simulink model "ES205_lab_5_dual_model_orig"  (R2021a)
settings: Solver=VariableStepAuto  StartTime=0.0  StopTime=tf_double  MaxStep=maxstep  RelTol=tol  AbsTol=tol
values from neighbouring files (symbols this model uses):
  a1 = 3.49    [ES205_lab_5_script.m]
  a2 = 3.24    [ES205_lab_5_script.m]
  Aout1 = pi * (d1/2)^2    (= 0.0881413088873)    [ES205_lab_5_script.m]
  Aout2 = pi * (d2/2)^2    (= 0.0452389342117)    [ES205_lab_5_script.m]
  Atank1 = 22.94    [ES205_lab_5_script.m]
  Atank2 = 22.94    [ES205_lab_5_script.m]
  b2 = 0.5    [ES205_lab_5_script.m]
  Cd1_orig = 0.7    [ES205_lab_5_script.m]
  Cd2_orig = 0.7    [ES205_lab_5_script.m]
  g = 32.2 * 12    (= 386.4)    [ES205_lab_5_script.m]
  h1_0_double = h1data_double(1)    [ES205_lab_5_script.m]
  h2_0_double = h2data_double(2)    [ES205_lab_5_script.m]
settings Model: Creator=schimmer  LastModifiedBy=schimmer
settings DataIOCC: SaveOutput=off  SignalLogging=off  DSMLogging=off  SaveTime=off  ReturnWorkspaceOutputs=off  OutputOption=SpecifiedOutputTimes  OutputTimes=tdata_double

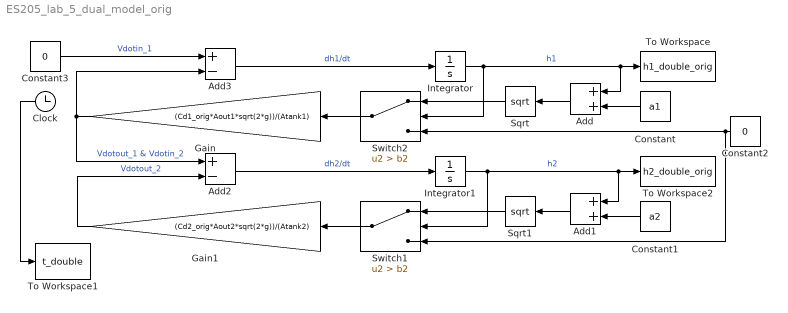
== system ES205_lab_5_dual_model_orig ==
  Add : Sum
  Add1 : Sum
  Add2 : Sum  Inputs=+-
  Add3 : Sum  Inputs=+-
  Clock : Clock
  Constant : Constant  Value=a1
  Constant1 : Constant  Value=a2
  Constant2 : Constant  Value=0
  Constant3 : Constant  Value=0
  Gain : Gain  Gain=(Cd1_orig*Aout1*sqrt(2*g))/(Atank1)
  Gain1 : Gain  Gain=(Cd2_orig*Aout2*sqrt(2*g))/(Atank2)
  Integrator : Integrator  InitialCondition=h1_0_double
  Integrator1 : Integrator  InitialCondition=h2_0_double
  Sqrt : Sqrt  SaturateOnIntegerOverflow=on
  Sqrt1 : Sqrt  SaturateOnIntegerOverflow=on
  Switch1 : Switch  Criteria=u2 > Threshold  Threshold=b2
  Switch2 : Switch  Criteria=u2 > Threshold  Threshold=b2
  To Workspace : ToWorkspace  VariableName=h1_double_orig  SampleTime=-1
  To Workspace1 : ToWorkspace  VariableName=t_double  SampleTime=-1
  To Workspace2 : ToWorkspace  VariableName=h2_double_orig  SampleTime=-1
  wires:
  Clock/1 -> To Workspace1/1
  Gain/1 -> Add2/1, Add3/2  "Vdotout_1 & Vdotin_2"
  Integrator/1 -> Add/1, To Workspace/1, Switch2/2  "h1"
  Sqrt/1 -> Switch2/1
  Add/1 -> Sqrt/1
  Constant/1 -> Add/2
  Constant1/1 -> Add1/2
  Integrator1/1 -> Switch1/2, Add1/1, To Workspace2/1  "h2"
  Add1/1 -> Sqrt1/1
  Switch2/1 -> Gain/1
  Add2/1 -> Integrator1/1  "dh2/dt"
  Sqrt1/1 -> Switch1/1
  Constant2/1 -> Switch1/3, Switch2/3
  Switch1/1 -> Gain1/1
  Constant3/1 -> Add3/1  "Vdotin_1"
  Add3/1 -> Integrator/1  "dh1/dt"
  Gain1/1 -> Add2/2  "Vdotout_2"
